simulink subsystem "Baseline"  (R2024b)
settings: Solver=VariableStepAuto  StartTime=0.0  StopTime=10.0  RelTol=1e-3
undefined symbols (not defined in the file or in its folder): SimIn, SimPar
libraries: simulink_extras x23, ComponentsLib x8, libAxisTransformations x3, AdaptiveLib x1
settings Model: Creator=tbritton  LastModifiedBy=mjki1
settings SolverCC: AlgebraicLoopSolver=TrustRegion
settings OptimizationCC: ReuseModelBlockBuffer=off
settings DebuggingCC: UnconnectedInputMsg=warning  UnconnectedOutputMsg=warning  UnconnectedLineMsg=warning
settings ModelReferenceCC: EnableRefExpFcnMdlSchedulingChecks=on
settings RTWCC: GPUComputeCapability=3.5  DLArmComputeVersion=19.05

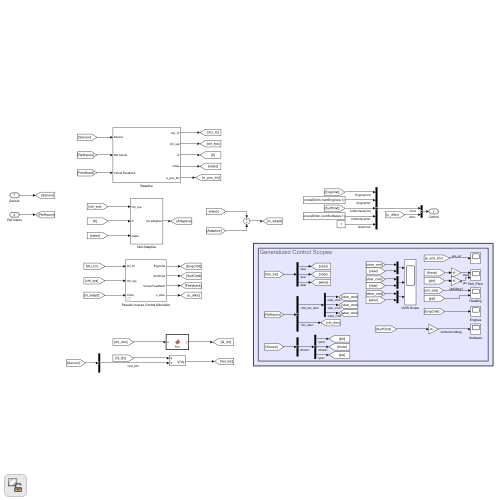
[thumbnail: Simulink's stored preview of the top-level diagram]
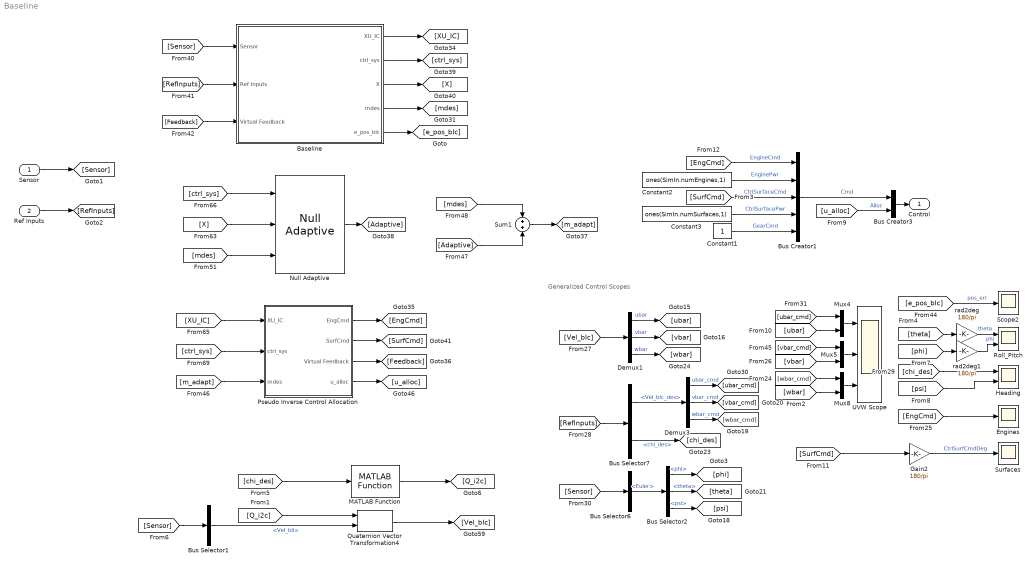
== system Baseline ==
  note: Generalized Control Scopes
  Sensor : Inport  OutDataTypeStr=Bus: SensorBus
  Ref Inputs : Inport  Port=2  OutDataTypeStr=Bus: BUS_REF_INPUT
  Baseline : Subsystem
      settings: LibrarySourceBlock=ControllersLib/Baseline
  Bus Creator1 : BusCreator  Inputs=5  OutDataTypeStr=Bus: BUS_CMD
  Bus Creator3 : BusCreator  Inputs=2
  Bus Selector1 : BusSelector  OutputSignals=Vel_bIi
  Bus Selector2 : BusSelector  OutputSignals=phi,theta,psi
  Bus Selector6 : BusSelector  OutputSignals=Euler
  Bus Selector7 : BusSelector  OutputSignals=Vel_bIc_des,chi_des
  Constant1 : Constant
  Constant2 : Constant  Value=ones(SimIn.numEngines,1)
  Constant3 : Constant  Value=ones(SimIn.numSurfaces,1)
  Demux1 : Demux  Outputs=3
  Demux3 : Demux  Outputs=3
  Engines : Scope
  Gain2 : Gain  Gain=180/pi
  Heading : Scope  NumInputPorts=2
  MATLAB Function : ComponentsLib/ConvertToControlFrame/MATLAB Function  SystemSampleTime=-1  VariantActivationTime=update diagram  AllowFlexibleInterface=on  Latency=0  AutoFrameSizeCalculation=off
      settings: SourceProductName=Components
  Mux4 : Mux  Inputs=2
  Mux5 : Mux  Inputs=2
  Mux8 : Mux  Inputs=2
  Null Adaptive : AdaptiveLib/Null Adaptive  SystemSampleTime=-1  VariantActivationTime=update diagram  AllowFlexibleInterface=on  Latency=0  AutoFrameSizeCalculation=off
      settings: SourceProductName=Adaptive Augmentation
  Pseudo Inverse Control Allocation : Subsystem  AncestorBlock=AllocatorsLib/Pseudo Inverse Control Allocation
      settings: LibrarySourceBlock=AllocatorsLib/Pseudo Inverse Control Allocation
  Quaternion Vector Transformation4 : libAxisTransformations/Quaternion Vector Transformation  n=0
  Roll_Pitch : Scope  NumInputPorts=2
  Scope2 : Scope
  Sum1 : Sum
  Surfaces : Scope
  UVW Scope : Scope  NumInputPorts=3
  rad2deg : Gain  Gain=180/pi
  rad2deg1 : Gain  Gain=180/pi
  Control : Outport  OutDataTypeStr=Bus: BUS_CONTROL  VectorParamsAs1DForOutWhenUnconnected=off
  wires:
  Baseline/5(e_pos_blc) -> [e_pos_bIc]
  Demux1/1 -> [ubar]  "ubar"
  Mux4/1 -> UVW Scope/1
  Demux3/3 -> [wbar_cmd]  "wbar_cmd"
  Mux5/1 -> UVW Scope/2
  [vbar_cmd] -> Mux5/1
  [ubar_cmd] -> Mux4/1
  [vbar] -> Mux5/2
  [SurfCmd] -> Gain2/1
  [chi_des] -> Heading/1
  [ubar] -> Mux4/2
  [Sensor] -> Bus Selector6/1
  [RefInputs] -> Bus Selector7/1
  [wbar] -> Mux8/2
  [phi] -> rad2deg1/1
  Demux3/2 -> [vbar_cmd]  "vbar_cmd"
  [e_pos_bIc] -> Scope2/1  "pos_err"
  Bus Selector6/1 -> Bus Selector2/1  "<Euler>"
  Bus Selector2/1 -> [phi]  "<phi>"
  Mux8/1 -> UVW Scope/3
  Bus Selector2/3 -> [psi]  "<psi>"
  Gain2/1 -> Surfaces/1  "CtrlSurfCmdDeg"
  [theta] -> rad2deg/1
  Bus Selector2/2 -> [theta]  "<theta>"
  [psi] -> Heading/2
  Demux1/2 -> [vbar]  "vbar"
  [EngCmd] -> Engines/1
  Bus Selector7/1 -> Demux3/1  "<Vel_bIc_des>"
  Demux3/1 -> [ubar_cmd]  "ubar_cmd"
  [Vel_bIc] -> Demux1/1
  Bus Selector7/2 -> [chi_des]  "<chi_des>"
  [wbar_cmd] -> Mux8/1
  Demux1/3 -> [wbar]  "wbar"
  [Sensor] -> Bus Selector1/1
  MATLAB Function/1 -> [Q_i2c]
  Quaternion Vector Transformation4/1 -> [Vel_bIc]
  [chi_des] -> MATLAB Function/1
  [Q_i2c] -> Quaternion Vector Transformation4/1
  Bus Selector1/1 -> Quaternion Vector Transformation4/2  "<Vel_bIi>"
  [ctrl_sys] -> Pseudo Inverse Control Allocation/2(ctrl_sys)
  [XU_IC] -> Pseudo Inverse Control Allocation/1(XU_IC)
  Pseudo Inverse Control Allocation/4(u_alloc) -> [u_alloc]
  Pseudo Inverse Control Allocation/2(SurfCmd) -> [SurfCmd]
  [Adaptive] -> Sum1/2
  [mdes] -> Sum1/1
  Sum1/1 -> [m_adapt]
  Baseline/3(X) -> [X]
  Baseline/2(ctrl_sys) -> [ctrl_sys]
  Null Adaptive/1 -> [Adaptive]
  [X] -> Null Adaptive/2
  [mdes] -> Null Adaptive/3
  [ctrl_sys] -> Null Adaptive/1
  Pseudo Inverse Control Allocation/1(EngCmd) -> [EngCmd]
  Baseline/1(XU_IC) -> [XU_IC]
  Pseudo Inverse Control Allocation/3(Virtual Feedback) -> [Feedback]
  [m_adapt] -> Pseudo Inverse Control Allocation/3(mdes)
  Baseline/4(mdes) -> [mdes]
  [Feedback] -> Baseline/3(Virtual Feedback)
  [RefInputs] -> Baseline/2(Ref Inputs)
  [Sensor] -> Baseline/1(Sensor)
  Constant3/1 -> Bus Creator1/4  "CtrlSurfacePwr"
  Constant2/1 -> Bus Creator1/2  "EnginePwr"
  [EngCmd] -> Bus Creator1/1  "EngineCmd"
  Sensor/1 -> [Sensor]
  Bus Creator1/1 -> Bus Creator3/1  "Cmd"
  [SurfCmd] -> Bus Creator1/3  "CtrlSurfaceCmd"
  Constant1/1 -> Bus Creator1/5  "GearCmd"
  Bus Creator3/1 -> Control/1
  [u_alloc] -> Bus Creator3/2  "Alloc"
  Ref Inputs/1 -> [RefInputs]
  rad2deg/1 -> Roll_Pitch/1  "theta"
  rad2deg1/1 -> Roll_Pitch/2  "phi"

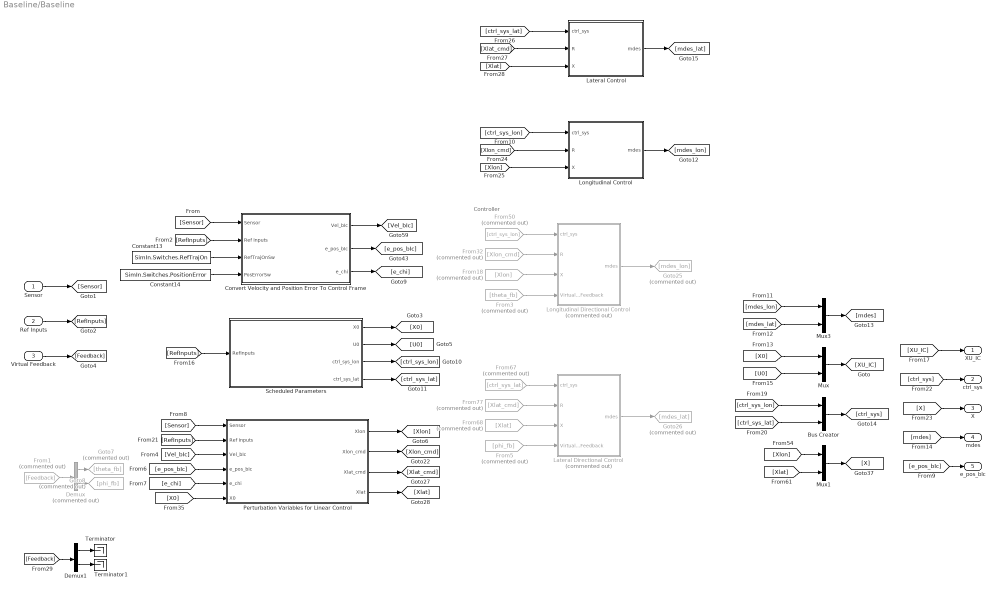
== system Baseline/Baseline ==
  note: Controller
  Sensor : Inport  OutDataTypeStr=Bus: SensorBus
  Ref Inputs : Inport  Port=2  OutDataTypeStr=Bus: BUS_REF_INPUT
  Virtual Feedback : Inport  Port=3
  Bus Creator : BusCreator  Inputs=2
  Constant13 : Constant  Value=SimIn.Switches.RefTrajOn
  Constant14 : Constant  Value=SimIn.Switches.PositionError
  Convert Velocity and Position Error To Control Frame : Subsystem  AncestorBlock=ComponentsLib/ConvertToControlFrame
  Demux : Demux  Commented=on  Outputs=2
  Demux1 : Demux  Outputs=2
  From1 : From  Commented=on  GotoTag=Feedback
  From18 : From  Commented=on  GotoTag=Xlon
  From3 : From  Commented=on  GotoTag=theta_fb
  From32 : From  Commented=on  GotoTag=Xlon_cmd
  From5 : From  Commented=on  GotoTag=phi_fb
  From50 : From  Commented=on  GotoTag=ctrl_sys_lon
  From67 : From  Commented=on  GotoTag=ctrl_sys_lat
  From68 : From  Commented=on  GotoTag=Xlat
  From77 : From  Commented=on  GotoTag=Xlat_cmd
  Goto25 : Goto  Commented=on  GotoTag=mdes_lon
  Goto26 : Goto  Commented=on  GotoTag=mdes_lat
  Goto7 : Goto  Commented=on  GotoTag=theta_fb
  Goto8 : Goto  Commented=on  GotoTag=phi_fb
  Lateral Control : Subsystem
  Lateral Directional Control : Subsystem  Commented=on  AncestorBlock=ComponentsLib/DirectionalControl
  Longitudinal Control : Subsystem
  Longitudinal Directional Control : Subsystem  Commented=on  AncestorBlock=ComponentsLib/DirectionalControl
      settings: LibrarySourceBlock=ComponentsLib/DirectionalControl
  Mux : Mux  Inputs=2
  Mux1 : Mux  Inputs=2
  Mux3 : Mux  Inputs=2
  Perturbation Variables for Linear Control : Subsystem  AncestorBlock=ComponentsLib/ComputePerturbationVariables
  Scheduled Parameters : Subsystem  AncestorBlock=ComponentsLib/FeedbackScheduling
      settings: LibrarySourceBlock=ComponentsLib/FeedbackScheduling
  Terminator : Terminator
  Terminator1 : Terminator
  XU_IC : Outport
  ctrl_sys : Outport  Port=2
  X : Outport  Port=3
  mdes : Outport  Port=4
  e_pos_blc : Outport  Port=5
  wires:
  [ctrl_sys_lat] -> Lateral Control/1(ctrl_sys)
  [Xlat] -> Lateral Control/3(X)
  [Xlat_cmd] -> Lateral Control/2(R)
  Lateral Control/1(mdes) -> [mdes_lat]
  Longitudinal Control/1(mdes) -> [mdes_lon]
  [Xlon] -> Longitudinal Control/3(X)
  [Xlon_cmd] -> Longitudinal Control/2(R)
  [ctrl_sys_lon] -> Longitudinal Control/1(ctrl_sys)
  [X] -> X/1
  [Xlat] -> Mux1/2
  [Xlon] -> Mux1/1
  Mux1/1 -> [X]
  [ctrl_sys] -> ctrl_sys/1
  Bus Creator/1 -> [ctrl_sys]
  [ctrl_sys_lat] -> Bus Creator/2
  [ctrl_sys_lon] -> Bus Creator/1
  [XU_IC] -> XU_IC/1
  Mux/1 -> [XU_IC]
  [U0] -> Mux/2
  [X0] -> Mux/1
  [mdes] -> mdes/1
  Mux3/1 -> [mdes]
  [mdes_lon] -> Mux3/1
  From5/1 -> Lateral Directional Control/4(Virtual Feedback)
  From3/1 -> Longitudinal Directional Control/4(Virtual Feedback)
  Demux/1 -> Goto7/1
  Demux/2 -> Goto8/1
  From1/1 -> Demux/1
  Virtual Feedback/1 -> [Feedback]
  From77/1 -> Lateral Directional Control/2(R)
  From18/1 -> Longitudinal Directional Control/3(X)
  From68/1 -> Lateral Directional Control/3(X)
  Longitudinal Directional Control/1(mdes) -> Goto25/1
  From50/1 -> Longitudinal Directional Control/1(ctrl_sys)
  From67/1 -> Lateral Directional Control/1(ctrl_sys)
  Lateral Directional Control/1(mdes) -> Goto26/1
  From32/1 -> Longitudinal Directional Control/2(R)
  Scheduled Parameters/4(ctrl_sys_lat) -> [ctrl_sys_lat]
  Scheduled Parameters/2(U0) -> [U0]
  [e_chi] -> Perturbation Variables for Linear Control/5(e_chi)
  Constant14/1 -> Convert Velocity and Position Error To Control Frame/4(PosErrorSw)
  [RefInputs] -> Perturbation Variables for Linear Control/2(Ref Inputs)
  Constant13/1 -> Convert Velocity and Position Error To Control Frame/3(RefTrajOnSw)
  [Vel_bIc] -> Perturbation Variables for Linear Control/3(Vel_bIc)
  [Sensor] -> Convert Velocity and Position Error To Control Frame/1(Sensor)
  Convert Velocity and Position Error To Control Frame/3(e_chi) -> [e_chi]
  Perturbation Variables for Linear Control/2(Xlon_cmd) -> [Xlon_cmd]
  [RefInputs] -> Scheduled Parameters/1(RefInputs)
  Perturbation Variables for Linear Control/4(Xlat) -> [Xlat]
  [e_pos_bIc] -> Perturbation Variables for Linear Control/4(e_pos_bIc)
  Scheduled Parameters/3(ctrl_sys_lon) -> [ctrl_sys_lon]
  Convert Velocity and Position Error To Control Frame/2(e_pos_bIc) -> [e_pos_bIc]
  Convert Velocity and Position Error To Control Frame/1(Vel_bIc) -> [Vel_bIc]
  [RefInputs] -> Convert Velocity and Position Error To Control Frame/2(Ref Inputs)
  Ref Inputs/1 -> [RefInputs]
  Scheduled Parameters/1(X0) -> [X0]
  Sensor/1 -> [Sensor]
  Perturbation Variables for Linear Control/3(Xlat_cmd) -> [Xlat_cmd]
  [Sensor] -> Perturbation Variables for Linear Control/1(Sensor)
  Perturbation Variables for Linear Control/1(Xlon) -> [Xlon]
  [X0] -> Perturbation Variables for Linear Control/6(X0)
  [e_pos_bIc] -> e_pos_blc/1
  [mdes_lat] -> Mux3/2
  Demux1/2 -> Terminator1/1
  [Feedback] -> Demux1/1
  Demux1/1 -> Terminator/1

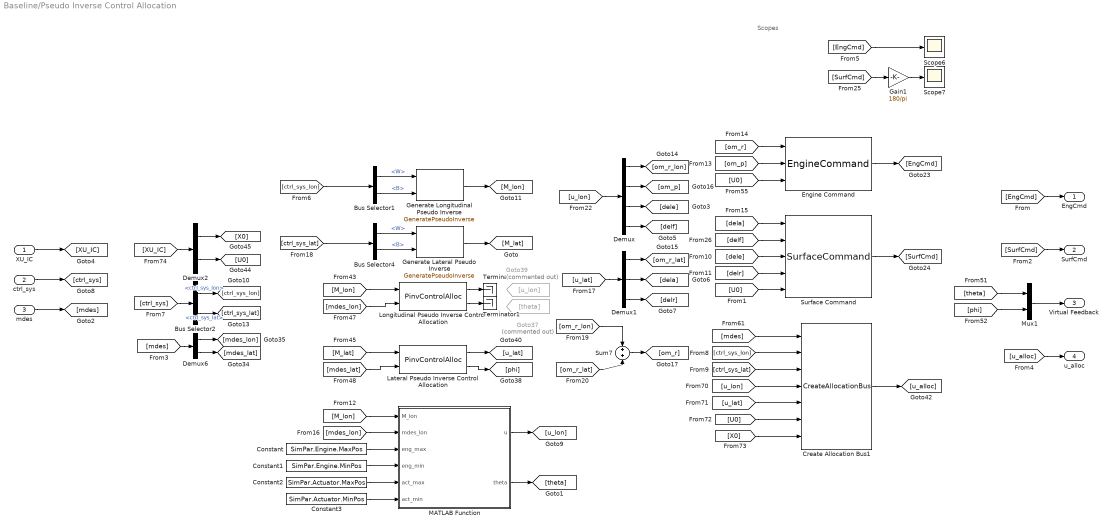
== system Baseline/Pseudo Inverse Control Allocation ==
  note: Scopes
  XU_IC : Inport
  ctrl_sys : Inport  Port=2
  mdes : Inport  Port=3
  Bus Selector1 : BusSelector  OutputSignals=W,B
  Bus Selector2 : BusSelector  OutputSignals=ctrl_sys_lon,ctrl_sys_lat
  Bus Selector4 : BusSelector  OutputSignals=W,B
  Constant : Constant  Value=SimPar.Engine.MaxPos
  Constant1 : Constant  Value=SimPar.Engine.MinPos
  Constant2 : Constant  Value=SimPar.Actuator.MaxPos
  Constant3 : Constant  Value=SimPar.Actuator.MinPos
  Create Allocation Bus1 : ComponentsLib/CreateAllocationBus  SystemSampleTime=-1  VariantActivationTime=update diagram  AllowFlexibleInterface=on  Latency=0  AutoFrameSizeCalculation=off
      settings: SourceProductName=Components
  Demux : Demux  Outputs=[8 1 1 1]
  Demux1 : Demux  Outputs=[8 1 1]
  Demux2 : Demux  Outputs=[12 13]
  Demux6 : Demux  Outputs=[3 3]
  Engine Command : ComponentsLib/EngineCommand  SystemSampleTime=-1  VariantActivationTime=update diagram  AllowFlexibleInterface=on  Latency=0  AutoFrameSizeCalculation=off
      settings: SourceProductName=Components
  Gain1 : Gain  Gain=180/pi
  Generate Lateral Pseudo Inverse : ComponentsLib/GeneratePseudoInverse  SystemSampleTime=-1  VariantActivationTime=update diagram  AllowFlexibleInterface=on  Latency=0  AutoFrameSizeCalculation=off
      settings: SourceProductName=Components
  Generate Longitudinal Pseudo Inverse : ComponentsLib/GeneratePseudoInverse  SystemSampleTime=-1  VariantActivationTime=update diagram  AllowFlexibleInterface=on  Latency=0  AutoFrameSizeCalculation=off
      settings: SourceProductName=Components
  Goto37 : Goto  Commented=on  GotoTag=theta
  Goto39 : Goto  Commented=on  GotoTag=u_lon
  Lateral Pseudo Inverse Control Allocation : ComponentsLib/PinvControlAlloc  SystemSampleTime=-1  VariantActivationTime=update diagram  AllowFlexibleInterface=on  Latency=0  AutoFrameSizeCalculation=off
      settings: SourceProductName=Components
  Longitudinal Pseudo Inverse Control Allocation : ComponentsLib/PinvControlAlloc  SystemSampleTime=-1  VariantActivationTime=update diagram  AllowFlexibleInterface=on  Latency=0  AutoFrameSizeCalculation=off
      settings: SourceProductName=Components
  MATLAB Function : MATLAB Function  TreatAsAtomicUnit=on
  Mux1 : Mux  Inputs=2
  Scope6 : Scope
  Scope7 : Scope
  Sum7 : Sum
  Surface Command : ComponentsLib/SurfaceCommand  SystemSampleTime=-1  VariantActivationTime=update diagram  AllowFlexibleInterface=on  Latency=0  AutoFrameSizeCalculation=off
      settings: SourceProductName=Components
  Terminator : Terminator
  Terminator1 : Terminator
  EngCmd : Outport
  SurfCmd : Outport  Port=2
  Virtual Feedback : Outport  Port=3
  u_alloc : Outport  Port=4
  wires:
  Constant/1 -> MATLAB Function/3(eng_max)
  Constant1/1 -> MATLAB Function/4(eng_min)
  Constant2/1 -> MATLAB Function/5(act_max)
  Constant3/1 -> MATLAB Function/6(act_min)
  MATLAB Function/2(theta) -> [theta]
  MATLAB Function/1(u) -> [u_lon]
  [mdes_lon] -> MATLAB Function/2(mdes_lon)
  [M_lon] -> MATLAB Function/1(M_lon)
  [ctrl_sys_lat] -> Create Allocation Bus1/3
  [ctrl_sys_lon] -> Create Allocation Bus1/2
  Bus Selector2/2 -> [ctrl_sys_lat]  "<ctrl_sys_lat>"
  Bus Selector2/1 -> [ctrl_sys_lon]  "<ctrl_sys_lon>"
  [ctrl_sys] -> Bus Selector2/1
  Bus Selector1/2 -> Generate Longitudinal Pseudo Inverse/2  "<B>"
  Bus Selector4/2 -> Generate Lateral Pseudo Inverse/2  "<B>"
  Generate Lateral Pseudo Inverse/1 -> [M_lat]
  Bus Selector4/1 -> Generate Lateral Pseudo Inverse/1  "<W>"
  Generate Longitudinal Pseudo Inverse/1 -> [M_lon]
  [ctrl_sys_lon] -> Bus Selector1/1
  Bus Selector1/1 -> Generate Longitudinal Pseudo Inverse/1  "<W>"
  [ctrl_sys_lat] -> Bus Selector4/1
  [EngCmd] -> Scope6/1
  [SurfCmd] -> Gain1/1
  Gain1/1 -> Scope7/1
  [u_alloc] -> u_alloc/1
  ctrl_sys/1 -> [ctrl_sys]
  XU_IC/1 -> [XU_IC]
  mdes/1 -> [mdes]
  [mdes] -> Demux6/1
  Demux6/1 -> [mdes_lon]
  Demux6/2 -> [mdes_lat]
  [mdes] -> Create Allocation Bus1/1
  Demux2/1 -> [X0]
  [X0] -> Create Allocation Bus1/7
  [XU_IC] -> Demux2/1
  [u_lat] -> Create Allocation Bus1/5
  Create Allocation Bus1/1 -> [u_alloc]
  [u_lon] -> Create Allocation Bus1/4
  [U0] -> Create Allocation Bus1/6
  Demux2/2 -> [U0]
  [SurfCmd] -> SurfCmd/1
  [EngCmd] -> EngCmd/1
  [dela] -> Surface Command/1
  [U0] -> Surface Command/5
  [om_r] -> Engine Command/1
  [om_p] -> Engine Command/2
  [delr] -> Surface Command/4
  [delf] -> Surface Command/2
  [dele] -> Surface Command/3
  [U0] -> Engine Command/3
  Surface Command/1 -> [SurfCmd]
  Engine Command/1 -> [EngCmd]
  Demux1/3 -> [delr]
  Demux/4 -> [delf]
  Demux/1 -> [om_r_lon]
  Demux1/1 -> [om_r_lat]
  Demux1/2 -> [dela]
  [u_lon] -> Demux/1
  Sum7/1 -> [om_r]
  [om_r_lon] -> Sum7/1
  [om_r_lat] -> Sum7/2
  [u_lat] -> Demux1/1
  Demux/2 -> [om_p]
  Demux/3 -> [dele]
  [M_lat] -> Lateral Pseudo Inverse Control Allocation/1
  [M_lon] -> Longitudinal Pseudo Inverse Control Allocation/1
  Mux1/1 -> Virtual Feedback/1
  Longitudinal Pseudo Inverse Control Allocation/2 -> Terminator1/1
  Lateral Pseudo Inverse Control Allocation/1 -> [u_lat]
  [mdes_lon] -> Longitudinal Pseudo Inverse Control Allocation/2
  [phi] -> Mux1/2
  [mdes_lat] -> Lateral Pseudo Inverse Control Allocation/2
  [theta] -> Mux1/1
  Longitudinal Pseudo Inverse Control Allocation/1 -> Terminator/1
  Lateral Pseudo Inverse Control Allocation/2 -> [phi]

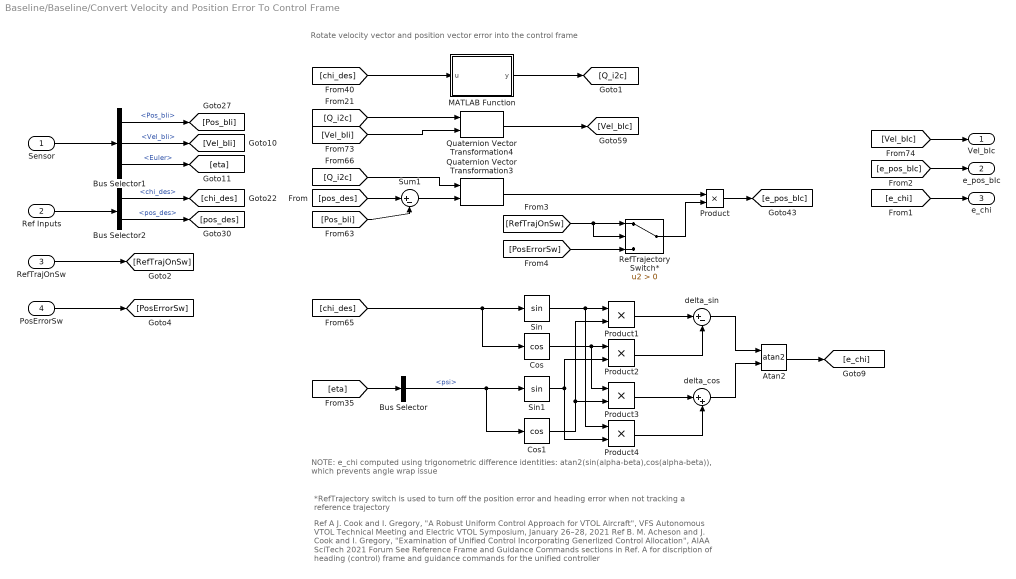
== system Baseline/Baseline/Convert Velocity and Position Error To Control Frame ==
  note: Rotate velocity vector and position vector error into the control frame
  note: Ref A
      | J. Cook and I. Gregory, "A Robust Uniform Control Approach for VTOL Aircraft", VFS Autonomous VTOL Technical Meeting and Electric VTOL Symposium, January 26–28, 2021
      |
      | Ref B.
      | M. Acheson and J. Cook and I. Gregory, "Examination of Unified Control Incorporating Generlized Control Allocation", AIAA SciTech 2021 Forum
      |
      | See Reference Frame and Guidance Commands sections in Ref. A for discription of heading (control) frame and guidance commands for the unified controller
  note: *RefTrajectory switch is used to turn off the position error and heading error when not tracking a reference trajectory
  note: NOTE: e_chi computed using trigonometric difference identities: atan2(sin(alpha-beta),cos(alpha-beta)), which prevents angle wrap issue
  Sensor : Inport  OutDataTypeStr=Bus: SensorBus
  Ref Inputs : Inport  Port=2  OutDataTypeStr=Bus: BUS_REF_INPUT
  RefTrajOnSw : Inport  Port=3
  PosErrorSw : Inport  Port=4
  Atan2 : Trigonometry  Operator=atan2
  Bus Selector : BusSelector  OutputSignals=psi
  Bus Selector1 : BusSelector  OutputSignals=Pos_bIi,Vel_bIi,Euler
  Bus Selector2 : BusSelector  OutputSignals=chi_des,pos_des
  Cos : Trigonometry  Operator=cos
  Cos1 : Trigonometry  Operator=cos
  MATLAB Function : MATLAB Function  TreatAsAtomicUnit=on
  Product{,1..4} (5 alike) : Product
  Quaternion Vector Transformation3 : libAxisTransformations/Quaternion Vector Transformation  n=0
  Quaternion Vector Transformation4 : libAxisTransformations/Quaternion Vector Transformation  n=0
  RefTrajectory Switch* : Switch  Criteria=u2 > Threshold  SaturateOnIntegerOverflow=off  InputSameDT=off
  Sin : Trigonometry
  Sin1 : Trigonometry
  Sum1 : Sum  Inputs=|+-
  delta_cos : Sum  Inputs=|++
  delta_sin : Sum  Inputs=|+-
  Vel_bIc : Outport
  e_pos_bIc : Outport  Port=2
  e_chi : Outport  Port=3
  wires:
  delta_cos/1 -> Atan2/2
  delta_sin/1 -> Atan2/1
  Product4/1 -> delta_cos/2
  Product3/1 -> delta_cos/1
  Product2/1 -> delta_sin/2
  Product1/1 -> delta_sin/1
  Cos1/1 -> Product1/2, Product3/2
  Sin1/1 -> Product2/2, Product4/2
  Cos/1 -> Product2/1, Product3/1
  Sin/1 -> Product4/1, Product1/1
  Bus Selector/1 -> Sin1/1, Cos1/1  "<psi>"
  [Q_i2c] -> Quaternion Vector Transformation4/1
  [eta] -> Bus Selector/1
  [PosErrorSw] -> RefTrajectory Switch*/3
  Bus Selector1/3 -> [eta]  "<Euler>"
  MATLAB Function/1(y) -> [Q_i2c]
  Ref Inputs/1 -> Bus Selector2/1
  Product/1 -> [e_pos_bIc]
  [Q_i2c] -> Quaternion Vector Transformation3/1
  Quaternion Vector Transformation3/1 -> Product/1
  [pos_des] -> Sum1/1
  [e_chi] -> e_chi/1
  [chi_des] -> MATLAB Function/1(u)
  RefTrajectory Switch*/1 -> Product/2
  [Pos_bIi] -> Sum1/2
  [Vel_bIc] -> Vel_bIc/1
  [RefTrajOnSw] -> RefTrajectory Switch*/2, RefTrajectory Switch*/1
  Bus Selector2/2 -> [pos_des]  "<pos_des>"
  Bus Selector1/1 -> [Pos_bIi]  "<Pos_bIi>"
  Atan2/1 -> [e_chi]
  [Vel_bIi] -> Quaternion Vector Transformation4/2
  PosErrorSw/1 -> [PosErrorSw]
  Bus Selector1/2 -> [Vel_bIi]  "<Vel_bIi>"
  Bus Selector2/1 -> [chi_des]  "<chi_des>"
  RefTrajOnSw/1 -> [RefTrajOnSw]
  [e_pos_bIc] -> e_pos_bIc/1
  Sum1/1 -> Quaternion Vector Transformation3/2
  [chi_des] -> Sin/1, Cos/1
  Quaternion Vector Transformation4/1 -> [Vel_bIc]
  Sensor/1 -> Bus Selector1/1

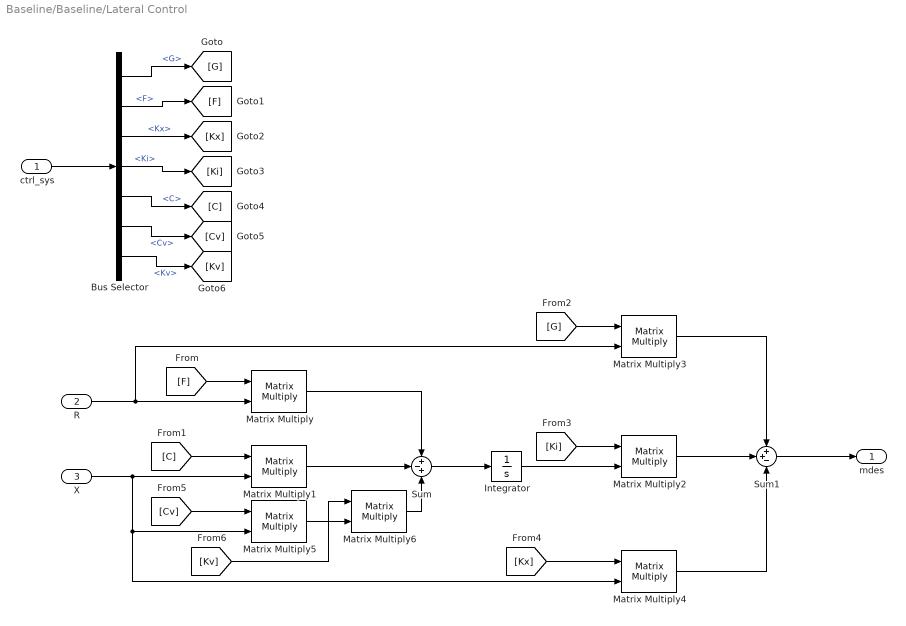
== system Baseline/Baseline/Lateral Control ==
  ctrl_sys : Inport
  R : Inport  Port=2
  X : Inport  Port=3
  Bus Selector : BusSelector  OutputSignals=G,F,Kx,Ki,C,Cv,Kv
  Integrator : Integrator
  Matrix Multiply{,1..6} (7 alike) : Product  Multiplication=Matrix(*)
  Sum : Sum  Inputs=+-+
  Sum1 : Sum  Inputs=++-
  mdes : Outport
  wires:
  Matrix Multiply6/1 -> Sum/3
  Matrix Multiply5/1 -> Matrix Multiply6/2
  [Kv] -> Matrix Multiply6/1
  [Cv] -> Matrix Multiply5/1
  Bus Selector/7 -> [Kv]  "<Kv>"
  Bus Selector/6 -> [Cv]  "<Cv>"
  Sum1/1 -> mdes/1
  Matrix Multiply4/1 -> Sum1/3
  [Kx] -> Matrix Multiply4/1
  Matrix Multiply2/1 -> Sum1/2
  Matrix Multiply3/1 -> Sum1/1
  [G] -> Matrix Multiply3/1
  Integrator/1 -> Matrix Multiply2/2
  Sum/1 -> Integrator/1
  [Ki] -> Matrix Multiply2/1
  Matrix Multiply/1 -> Sum/1
  Matrix Multiply1/1 -> Sum/2
  X/1 -> Matrix Multiply4/2, Matrix Multiply5/2, Matrix Multiply1/2
  [C] -> Matrix Multiply1/1
  [F] -> Matrix Multiply/1
  R/1 -> Matrix Multiply/2, Matrix Multiply3/2
  Bus Selector/5 -> [C]  "<C>"
  Bus Selector/4 -> [Ki]  "<Ki>"
  Bus Selector/3 -> [Kx]  "<Kx>"
  Bus Selector/2 -> [F]  "<F>"
  Bus Selector/1 -> [G]  "<G>"
  ctrl_sys/1 -> Bus Selector/1

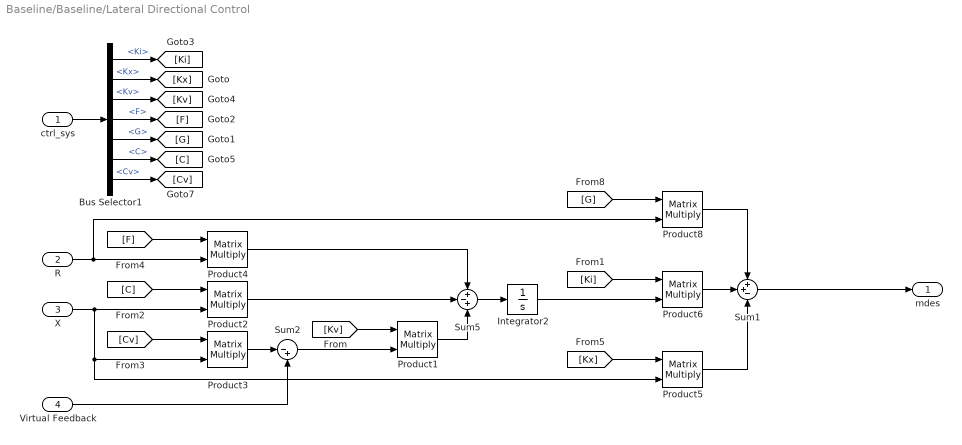
== system Baseline/Baseline/Lateral Directional Control ==
  ctrl_sys : Inport
  R : Inport  Port=2
  X : Inport  Port=3
  Virtual Feedback : Inport  Port=4
  Bus Selector1 : BusSelector  OutputSignals=Ki,Kx,Kv,F,G,C,Cv
  Integrator2 : Integrator  UpperSaturationLimit=[10 10 1]  LowerSaturationLimit=[-10 -10 -1]
  Product{1..6,8} (7 alike) : Product  Multiplication=Matrix(*)
  Sum1 : Sum  Inputs=++-
  Sum2 : Sum  Inputs=|-+
  Sum5 : Sum  Inputs=+-+
  mdes : Outport
  wires:
  Bus Selector1/1 -> [Ki]  "<Ki>"
  Bus Selector1/2 -> [Kx]  "<Kx>"
  Bus Selector1/3 -> [Kv]  "<Kv>"
  Bus Selector1/4 -> [F]  "<F>"
  Bus Selector1/5 -> [G]  "<G>"
  Bus Selector1/6 -> [C]  "<C>"
  Bus Selector1/7 -> [Cv]  "<Cv>"
  Virtual Feedback/1 -> Sum2/2
  [G] -> Product8/1
  Product8/1 -> Sum1/1
  Product4/1 -> Sum5/1
  [F] -> Product4/1
  Product5/1 -> Sum1/3
  [Kx] -> Product5/1
  Product6/1 -> Sum1/2
  [Ki] -> Product6/1
  Product1/1 -> Sum5/3
  [Kv] -> Product1/1
  Sum2/1 -> Product1/2
  Integrator2/1 -> Product6/2
  Product3/1 -> Sum2/1
  [Cv] -> Product3/1
  ctrl_sys/1 -> Bus Selector1/1
  Sum5/1 -> Integrator2/1
  R/1 -> Product4/2, Product8/2
  Product2/1 -> Sum5/2
  [C] -> Product2/1
  X/1 -> Product5/2, Product3/2, Product2/2
  Sum1/1 -> mdes/1

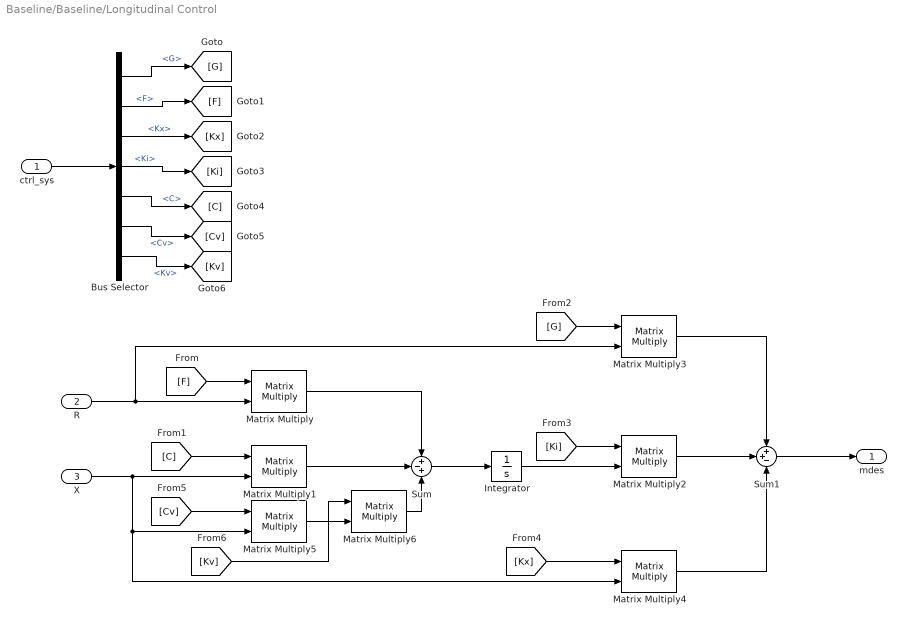
== system Baseline/Baseline/Longitudinal Control ==
  ctrl_sys : Inport
  R : Inport  Port=2
  X : Inport  Port=3
  Bus Selector : BusSelector  OutputSignals=G,F,Kx,Ki,C,Cv,Kv
  Integrator : Integrator
  Matrix Multiply{,1..6} (7 alike) : Product  Multiplication=Matrix(*)
  Sum : Sum  Inputs=+-+
  Sum1 : Sum  Inputs=++-
  mdes : Outport
  wires:
  Bus Selector/7 -> [Kv]  "<Kv>"
  Bus Selector/2 -> [F]  "<F>"
  Bus Selector/1 -> [G]  "<G>"
  [C] -> Matrix Multiply1/1
  Matrix Multiply3/1 -> Sum1/1
  Sum1/1 -> mdes/1
  [F] -> Matrix Multiply/1
  [Kv] -> Matrix Multiply6/1
  Bus Selector/5 -> [C]  "<C>"
  Sum/1 -> Integrator/1
  [G] -> Matrix Multiply3/1
  Integrator/1 -> Matrix Multiply2/2
  Matrix Multiply2/1 -> Sum1/2
  Matrix Multiply1/1 -> Sum/2
  Bus Selector/4 -> [Ki]  "<Ki>"
  Matrix Multiply6/1 -> Sum/3
  R/1 -> Matrix Multiply/2, Matrix Multiply3/2
  Matrix Multiply/1 -> Sum/1
  [Kx] -> Matrix Multiply4/1
  Matrix Multiply5/1 -> Matrix Multiply6/2
  Bus Selector/3 -> [Kx]  "<Kx>"
  X/1 -> Matrix Multiply4/2, Matrix Multiply5/2, Matrix Multiply1/2
  Matrix Multiply4/1 -> Sum1/3
  [Ki] -> Matrix Multiply2/1
  [Cv] -> Matrix Multiply5/1
  ctrl_sys/1 -> Bus Selector/1
  Bus Selector/6 -> [Cv]  "<Cv>"

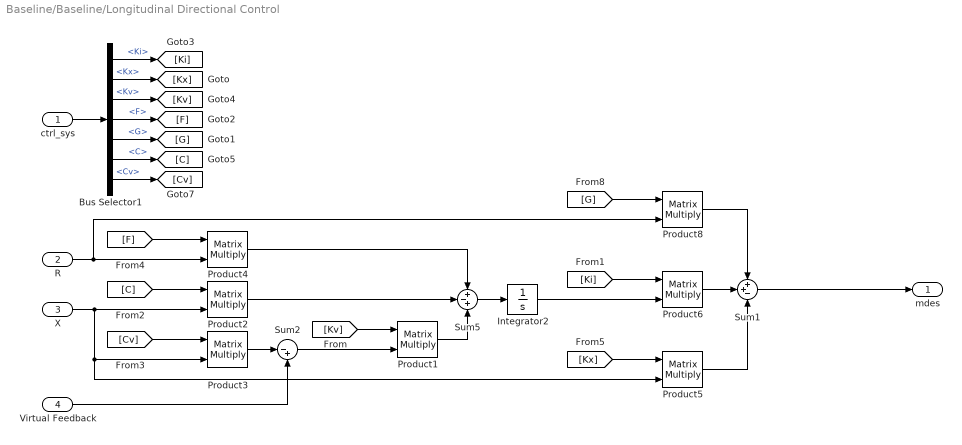
== system Baseline/Baseline/Longitudinal Directional Control ==
  ctrl_sys : Inport
  R : Inport  Port=2
  X : Inport  Port=3
  Virtual Feedback : Inport  Port=4
  Bus Selector1 : BusSelector  OutputSignals=Ki,Kx,Kv,F,G,C,Cv
  Integrator2 : Integrator  UpperSaturationLimit=[10 10 1]  LowerSaturationLimit=[-10 -10 -1]
  Product{1..6,8} (7 alike) : Product  Multiplication=Matrix(*)
  Sum1 : Sum  Inputs=++-
  Sum2 : Sum  Inputs=|-+
  Sum5 : Sum  Inputs=+-+
  mdes : Outport
  wires:
  Bus Selector1/1 -> [Ki]  "<Ki>"
  Bus Selector1/2 -> [Kx]  "<Kx>"
  Bus Selector1/3 -> [Kv]  "<Kv>"
  Bus Selector1/4 -> [F]  "<F>"
  Bus Selector1/5 -> [G]  "<G>"
  Bus Selector1/6 -> [C]  "<C>"
  Bus Selector1/7 -> [Cv]  "<Cv>"
  Virtual Feedback/1 -> Sum2/2
  [G] -> Product8/1
  Product8/1 -> Sum1/1
  Product4/1 -> Sum5/1
  [F] -> Product4/1
  Product5/1 -> Sum1/3
  [Kx] -> Product5/1
  Product6/1 -> Sum1/2
  [Ki] -> Product6/1
  Product1/1 -> Sum5/3
  [Kv] -> Product1/1
  Sum2/1 -> Product1/2
  Integrator2/1 -> Product6/2
  Product3/1 -> Sum2/1
  [Cv] -> Product3/1
  ctrl_sys/1 -> Bus Selector1/1
  Sum5/1 -> Integrator2/1
  R/1 -> Product4/2, Product8/2
  Product2/1 -> Sum5/2
  [C] -> Product2/1
  X/1 -> Product5/2, Product3/2, Product2/2
  Sum1/1 -> mdes/1

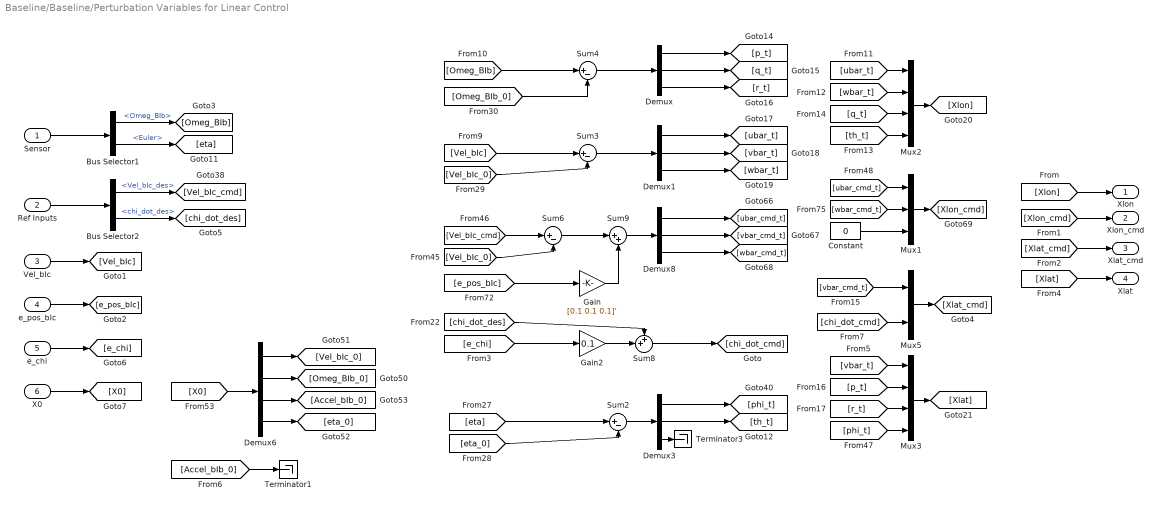
== system Baseline/Baseline/Perturbation Variables for Linear Control ==
  Sensor : Inport  OutDataTypeStr=Bus: SensorBus
  Ref Inputs : Inport  Port=2  OutDataTypeStr=Bus: BUS_REF_INPUT
  Vel_bIc : Inport  Port=3
  e_pos_bIc : Inport  Port=4
  e_chi : Inport  Port=5
  X0 : Inport  Port=6
  Bus Selector1 : BusSelector  OutputSignals=Omeg_BIb,Euler
  Bus Selector2 : BusSelector  OutputSignals=Vel_bIc_des,chi_dot_des
  Constant : Constant  Value=0
  Demux{,1,3,8} (4 alike) : Demux  Outputs=3
  Demux6 : Demux  Outputs=[3 3 3 3]
  Gain : Gain  Gain=[0.1 0.1 0.1]'
  Gain2 : Gain  Gain=0.1
  Mux1 : Mux  Inputs=3
  Mux2 : Mux
  Mux3 : Mux
  Mux5 : Mux  Inputs=2
  Sum{2..4,6} (4 alike) : Sum  Inputs=|+-
  Sum8 : Sum  Inputs=++|
  Sum9 : Sum  Inputs=|++
  Terminator1 : Terminator
  Terminator3 : Terminator
  Xlon : Outport
  Xlon_cmd : Outport  Port=2
  Xlat_cmd : Outport  Port=3
  Xlat : Outport  Port=4
  wires:
  [Accel_bIb_0] -> Terminator1/1
  X0/1 -> [X0]
  Demux6/2 -> [Omeg_BIb_0]
  Demux6/4 -> [eta_0]
  [X0] -> Demux6/1
  Demux6/3 -> [Accel_bIb_0]
  Demux6/1 -> [Vel_bIc_0]
  e_chi/1 -> [e_chi]
  e_pos_bIc/1 -> [e_pos_bIc]
  Bus Selector2/2 -> [chi_dot_des]  "<chi_dot_des>"
  Bus Selector2/1 -> [Vel_bIc_cmd]  "<Vel_bIc_des>"
  Ref Inputs/1 -> Bus Selector2/1
  Vel_bIc/1 -> [Vel_bIc]
  Bus Selector1/1 -> [Omeg_BIb]  "<Omeg_BIb>"
  Sensor/1 -> Bus Selector1/1
  Bus Selector1/2 -> [eta]  "<Euler>"
  [Xlat] -> Xlat/1
  [Xlat_cmd] -> Xlat_cmd/1
  [Xlon_cmd] -> Xlon_cmd/1
  [Xlon] -> Xlon/1
  [Omeg_BIb] -> Sum4/1
  [eta_0] -> Sum2/2
  [wbar_t] -> Mux2/2
  [ubar_cmd_t] -> Mux1/1
  Demux/2 -> [q_t]
  [th_t] -> Mux2/4
  [p_t] -> Mux3/2
  Mux3/1 -> [Xlat]
  Sum4/1 -> Demux/1
  Sum3/1 -> Demux1/1
  Demux/3 -> [r_t]
  Sum2/1 -> Demux3/1
  Demux8/2 -> [vbar_cmd_t]
  [Vel_bIc_cmd] -> Sum6/1
  Sum6/1 -> Sum9/1
  Demux8/1 -> [ubar_cmd_t]
  [phi_t] -> Mux3/4
  Constant/1 -> Mux1/3
  Demux8/3 -> [wbar_cmd_t]
  [e_pos_bIc] -> Gain/1
  [wbar_cmd_t] -> Mux1/2
  [vbar_t] -> Mux3/1
  Mux1/1 -> [Xlon_cmd]
  [chi_dot_des] -> Sum8/1
  Demux1/2 -> [vbar_t]
  [q_t] -> Mux2/3
  Mux5/1 -> [Xlat_cmd]
  [ubar_t] -> Mux2/1
  Gain/1 -> Sum9/2
  [vbar_cmd_t] -> Mux5/1
  [r_t] -> Mux3/3
  [Vel_bIc_0] -> Sum6/2
  [e_chi] -> Gain2/1
  Sum8/1 -> [chi_dot_cmd]
  Mux2/1 -> [Xlon]
  Gain2/1 -> Sum8/2
  Demux/1 -> [p_t]
  Demux1/3 -> [wbar_t]
  Demux3/1 -> [phi_t]
  Demux3/3 -> Terminator3/1
  Demux3/2 -> [th_t]
  [eta] -> Sum2/1
  Demux1/1 -> [ubar_t]
  [chi_dot_cmd] -> Mux5/2
  [Vel_bIc_0] -> Sum3/2
  [Vel_bIc] -> Sum3/1
  Sum9/1 -> Demux8/1
  [Omeg_BIb_0] -> Sum4/2

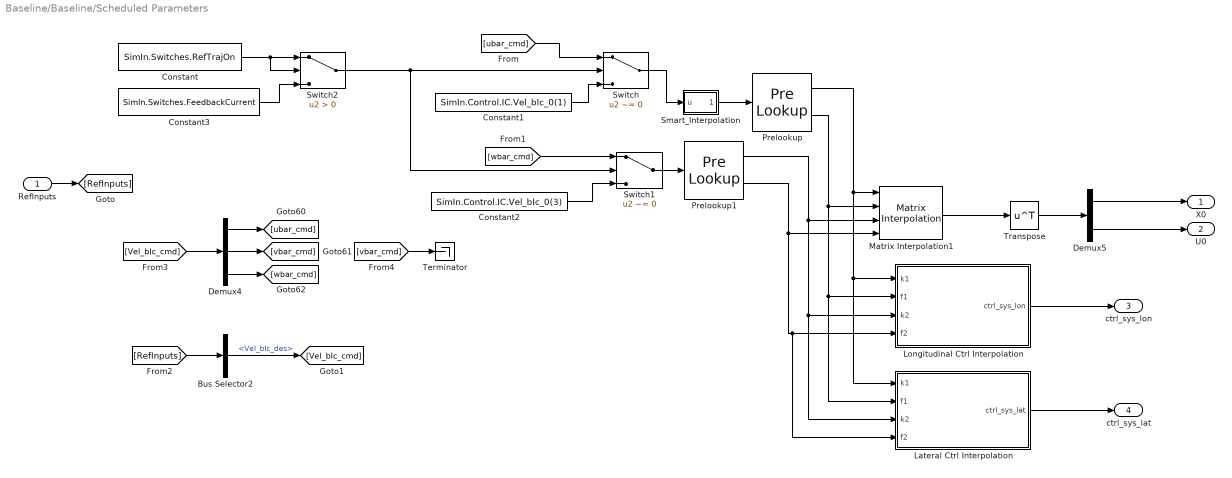
== system Baseline/Baseline/Scheduled Parameters ==
  RefInputs : Inport  OutDataTypeStr=Bus: BUS_REF_INPUT
  Bus Selector2 : BusSelector  OutputSignals=Vel_bIc_des
  Constant : Constant  Value=SimIn.Switches.RefTrajOn
  Constant1 : Constant  Value=SimIn.Control.IC.Vel_bIc_0(1)
  Constant2 : Constant  Value=SimIn.Control.IC.Vel_bIc_0(3)
  Constant3 : Constant  Value=SimIn.Switches.FeedbackCurrent
  Demux4 : Demux  Outputs=3
  Demux5 : Demux  Outputs=[12 13]
  Lateral Ctrl Interpolation : Subsystem
  Longitudinal Ctrl Interpolation : Subsystem
  Matrix Interpolation1 : simulink_extras/Additional Lookup Tables/Matrix Interpolation  InterpMethod=Linear  ExtrapMethod=Clip  InterpolateDimension=2  TableData=SimIn.Control.trim.XU0_interp  SimulateUsing=Code generation
  Prelookup : PreLookup  BreakpointsData=SimIn.Control.trim.UH
  Prelookup1 : PreLookup  BreakpointsData=SimIn.Control.trim.WH
  Smart_Interpolation : MATLAB Function  TreatAsAtomicUnit=on
  Switch : Switch  Criteria=u2 ~= 0  SaturateOnIntegerOverflow=off  InputSameDT=off
  Switch1 : Switch  Criteria=u2 ~= 0  SaturateOnIntegerOverflow=off  InputSameDT=off
  Switch2 : Switch  Criteria=u2 > Threshold  SaturateOnIntegerOverflow=off  InputSameDT=off
  Terminator : Terminator
  Transpose : Math  Operator=transpose
  X0 : Outport
  U0 : Outport  Port=2
  ctrl_sys_lon : Outport  Port=3
  ctrl_sys_lat : Outport  Port=4
  wires:
  [wbar_cmd] -> Switch1/1
  [vbar_cmd] -> Terminator/1
  Bus Selector2/1 -> [Vel_bIc_cmd]  "<Vel_bIc_des>"
  [RefInputs] -> Bus Selector2/1
  [ubar_cmd] -> Switch/1
  RefInputs/1 -> [RefInputs]
  [Vel_bIc_cmd] -> Demux4/1
  Demux4/2 -> [vbar_cmd]
  Demux4/3 -> [wbar_cmd]
  Demux4/1 -> [ubar_cmd]
  Matrix Interpolation1/1 -> Transpose/1
  Transpose/1 -> Demux5/1
  Demux5/1 -> X0/1
  Demux5/2 -> U0/1
  Prelookup1/1 -> Longitudinal Ctrl Interpolation/3(k2), Lateral Ctrl Interpolation/3(k2), Matrix Interpolation1/3
  Prelookup1/2 -> Longitudinal Ctrl Interpolation/4(f2), Lateral Ctrl Interpolation/4(f2), Matrix Interpolation1/4
  Lateral Ctrl Interpolation/1(ctrl_sys_lat) -> ctrl_sys_lat/1
  Longitudinal Ctrl Interpolation/1(ctrl_sys_lon) -> ctrl_sys_lon/1
  Constant1/1 -> Switch/3
  Switch1/1 -> Prelookup1/1
  Constant2/1 -> Switch1/3
  Switch2/1 -> Switch1/2, Switch/2
  Constant/1 -> Switch2/1, Switch2/2
  Constant3/1 -> Switch2/3
  Switch/1 -> Smart_Interpolation/1(u)
  Smart_Interpolation/1(u_out) -> Prelookup/1
  Prelookup/2 -> Longitudinal Ctrl Interpolation/2(f1), Lateral Ctrl Interpolation/2(f1), Matrix Interpolation1/2
  Prelookup/1 -> Matrix Interpolation1/1, Longitudinal Ctrl Interpolation/1(k1), Lateral Ctrl Interpolation/1(k1)

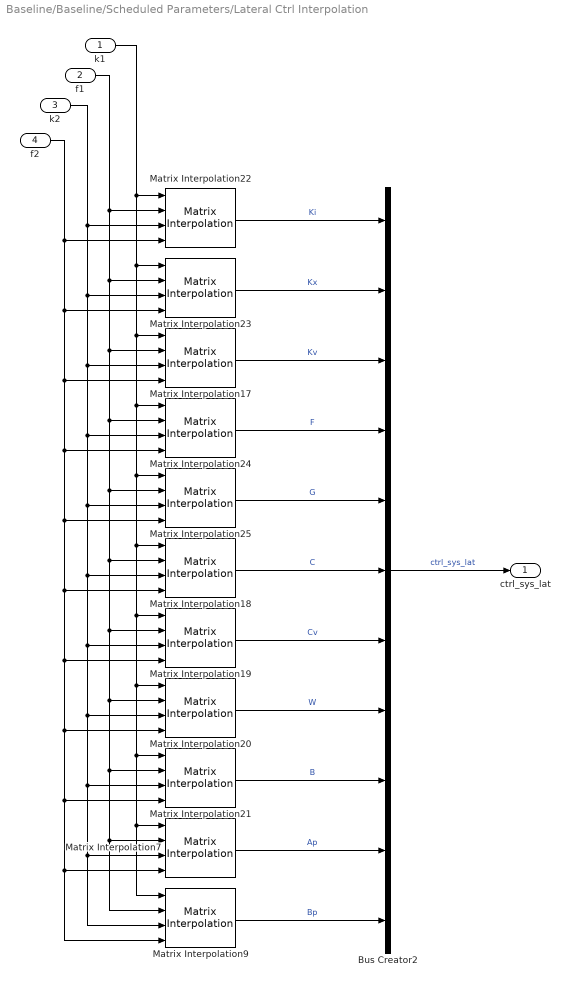
== system Baseline/Baseline/Scheduled Parameters/Lateral Ctrl Interpolation ==
  k1 : Inport
  f1 : Inport  Port=2
  k2 : Inport  Port=3
  f2 : Inport  Port=4
  Bus Creator2 : BusCreator  Inputs=11
  Matrix Interpolation17 : simulink_extras/Additional Lookup Tables/Matrix Interpolation  InterpMethod=Linear  ExtrapMethod=Clip  InterpolateDimension=2  TableData=SimIn.Control.trim.Kv_lat_interp  SimulateUsing=Code generation
  Matrix Interpolation18 : simulink_extras/Additional Lookup Tables/Matrix Interpolation  InterpMethod=Linear  ExtrapMethod=Clip  InterpolateDimension=2  TableData=SimIn.Control.trim.C_lat_interp  SimulateUsing=Code generation
  Matrix Interpolation19 : simulink_extras/Additional Lookup Tables/Matrix Interpolation  InterpMethod=Linear  ExtrapMethod=Clip  InterpolateDimension=2  TableData=SimIn.Control.trim.Cv_lat_interp  SimulateUsing=Code generation
  Matrix Interpolation20 : simulink_extras/Additional Lookup Tables/Matrix Interpolation  InterpMethod=Linear  ExtrapMethod=Clip  InterpolateDimension=2  TableData=SimIn.Control.trim.W_lat_interp  SimulateUsing=Code generation
  Matrix Interpolation21 : simulink_extras/Additional Lookup Tables/Matrix Interpolation  InterpMethod=Linear  ExtrapMethod=Clip  InterpolateDimension=2  TableData=SimIn.Control.trim.B_lat_interp  SimulateUsing=Code generation
  Matrix Interpolation22 : simulink_extras/Additional Lookup Tables/Matrix Interpolation  InterpMethod=Linear  ExtrapMethod=Clip  InterpolateDimension=2  TableData=SimIn.Control.trim.Ki_lat_interp  SimulateUsing=Code generation
  Matrix Interpolation23 : simulink_extras/Additional Lookup Tables/Matrix Interpolation  InterpMethod=Linear  ExtrapMethod=Clip  InterpolateDimension=2  TableData=SimIn.Control.trim.Kx_lat_interp  SimulateUsing=Code generation
  Matrix Interpolation24 : simulink_extras/Additional Lookup Tables/Matrix Interpolation  InterpMethod=Linear  ExtrapMethod=Clip  InterpolateDimension=2  TableData=SimIn.Control.trim.F_lat_interp  SimulateUsing=Code generation
  Matrix Interpolation25 : simulink_extras/Additional Lookup Tables/Matrix Interpolation  InterpMethod=Linear  ExtrapMethod=Clip  InterpolateDimension=2  TableData=SimIn.Control.trim.G_lat_interp  SimulateUsing=Code generation
  Matrix Interpolation7 : simulink_extras/Additional Lookup Tables/Matrix Interpolation  InterpMethod=Linear  ExtrapMethod=Clip  InterpolateDimension=2  TableData=SimIn.Control.trim.Ap_lat_interp  SimulateUsing=Code generation
  Matrix Interpolation9 : simulink_extras/Additional Lookup Tables/Matrix Interpolation  InterpMethod=Linear  ExtrapMethod=Clip  InterpolateDimension=2  TableData=SimIn.Control.trim.Bp_lat_interp  SimulateUsing=Code generation
  ctrl_sys_lat : Outport
  wires:
  k1/1 -> Matrix Interpolation22/1, Matrix Interpolation23/1, Matrix Interpolation17/1, Matrix Interpolation25/1, Matrix Interpolation18/1, Matrix Interpolation19/1, Matrix Interpolation21/1, Matrix Interpolation9/1, Matrix Interpolation7/1, Matrix Interpolation20/1, Matrix Interpolation24/1
  k2/1 -> Matrix Interpolation22/3, Matrix Interpolation23/3, Matrix Interpolation17/3, Matrix Interpolation24/3, Matrix Interpolation25/3, Matrix Interpolation18/3, Matrix Interpolation19/3, Matrix Interpolation20/3, Matrix Interpolation21/3, Matrix Interpolation7/3, Matrix Interpolation9/3
  Matrix Interpolation20/1 -> Bus Creator2/8  "W"
  f2/1 -> Matrix Interpolation22/4, Matrix Interpolation23/4, Matrix Interpolation17/4, Matrix Interpolation24/4, Matrix Interpolation25/4, Matrix Interpolation18/4, Matrix Interpolation19/4, Matrix Interpolation20/4, Matrix Interpolation21/4, Matrix Interpolation7/4, Matrix Interpolation9/4
  f1/1 -> Matrix Interpolation22/2, Matrix Interpolation23/2, Matrix Interpolation17/2, Matrix Interpolation24/2, Matrix Interpolation25/2, Matrix Interpolation18/2, Matrix Interpolation19/2, Matrix Interpolation20/2, Matrix Interpolation21/2, Matrix Interpolation7/2, Matrix Interpolation9/2
  Matrix Interpolation22/1 -> Bus Creator2/1  "Ki"
  Matrix Interpolation17/1 -> Bus Creator2/3  "Kv"
  Matrix Interpolation18/1 -> Bus Creator2/6  "C"
  Matrix Interpolation19/1 -> Bus Creator2/7  "Cv"
  Matrix Interpolation23/1 -> Bus Creator2/2  "Kx"
  Matrix Interpolation9/1 -> Bus Creator2/11  "Bp"
  Matrix Interpolation25/1 -> Bus Creator2/5  "G"
  Matrix Interpolation24/1 -> Bus Creator2/4  "F"
  Matrix Interpolation21/1 -> Bus Creator2/9  "B"
  Matrix Interpolation7/1 -> Bus Creator2/10  "Ap"
  Bus Creator2/1 -> ctrl_sys_lat/1  "ctrl_sys_lat"

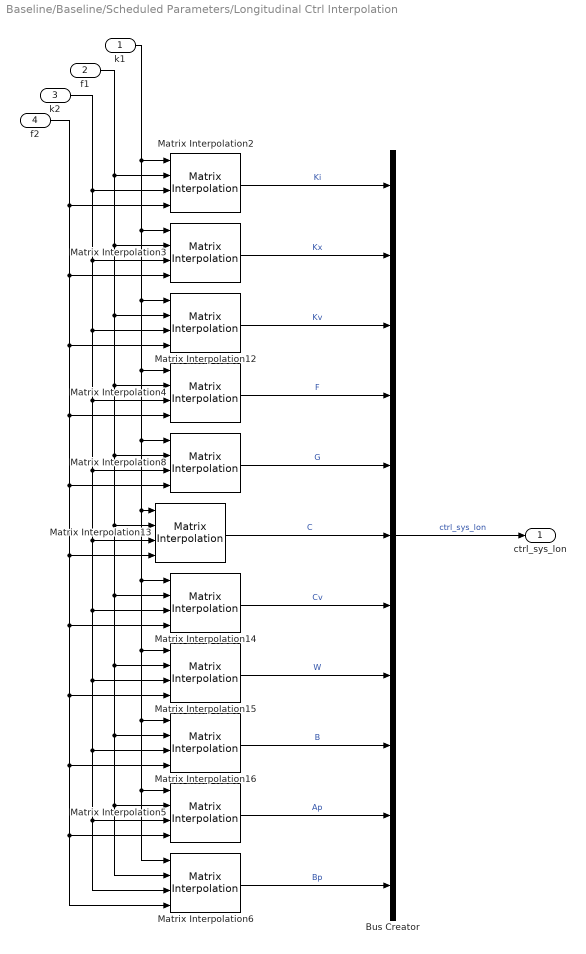
== system Baseline/Baseline/Scheduled Parameters/Longitudinal Ctrl Interpolation ==
  k1 : Inport
  f1 : Inport  Port=2
  k2 : Inport  Port=3
  f2 : Inport  Port=4
  Bus Creator : BusCreator  Inputs=11
  Matrix Interpolation12 : simulink_extras/Additional Lookup Tables/Matrix Interpolation  InterpMethod=Linear  ExtrapMethod=Clip  InterpolateDimension=2  TableData=SimIn.Control.trim.Kv_lon_interp  SimulateUsing=Code generation
  Matrix Interpolation13 : simulink_extras/Additional Lookup Tables/Matrix Interpolation  InterpMethod=Linear  ExtrapMethod=Clip  InterpolateDimension=2  TableData=SimIn.Control.trim.C_lon_interp  SimulateUsing=Code generation
  Matrix Interpolation14 : simulink_extras/Additional Lookup Tables/Matrix Interpolation  InterpMethod=Linear  ExtrapMethod=Clip  InterpolateDimension=2  TableData=SimIn.Control.trim.Cv_lon_interp  SimulateUsing=Code generation
  Matrix Interpolation15 : simulink_extras/Additional Lookup Tables/Matrix Interpolation  InterpMethod=Linear  ExtrapMethod=Clip  InterpolateDimension=2  TableData=SimIn.Control.trim.W_lon_interp  SimulateUsing=Code generation
  Matrix Interpolation16 : simulink_extras/Additional Lookup Tables/Matrix Interpolation  InterpMethod=Linear  ExtrapMethod=Clip  InterpolateDimension=2  TableData=SimIn.Control.trim.B_lon_interp  SimulateUsing=Code generation
  Matrix Interpolation2 : simulink_extras/Additional Lookup Tables/Matrix Interpolation  InterpMethod=Linear  ExtrapMethod=Clip  InterpolateDimension=2  TableData=SimIn.Control.trim.Ki_lon_interp  SimulateUsing=Code generation
  Matrix Interpolation3 : simulink_extras/Additional Lookup Tables/Matrix Interpolation  InterpMethod=Linear  ExtrapMethod=Clip  InterpolateDimension=2  TableData=SimIn.Control.trim.Kx_lon_interp  SimulateUsing=Code generation
  Matrix Interpolation4 : simulink_extras/Additional Lookup Tables/Matrix Interpolation  InterpMethod=Linear  ExtrapMethod=Clip  InterpolateDimension=2  TableData=SimIn.Control.trim.F_lon_interp  SimulateUsing=Code generation
  Matrix Interpolation5 : simulink_extras/Additional Lookup Tables/Matrix Interpolation  InterpMethod=Linear  ExtrapMethod=Clip  InterpolateDimension=2  TableData=SimIn.Control.trim.Ap_lon_interp  SimulateUsing=Code generation
  Matrix Interpolation6 : simulink_extras/Additional Lookup Tables/Matrix Interpolation  InterpMethod=Linear  ExtrapMethod=Clip  InterpolateDimension=2  TableData=SimIn.Control.trim.Bp_lon_interp  SimulateUsing=Code generation
  Matrix Interpolation8 : simulink_extras/Additional Lookup Tables/Matrix Interpolation  InterpMethod=Linear  ExtrapMethod=Clip  InterpolateDimension=2  TableData=SimIn.Control.trim.G_lon_interp  SimulateUsing=Code generation
  ctrl_sys_lon : Outport
  wires:
  f1/1 -> Matrix Interpolation2/2, Matrix Interpolation3/2, Matrix Interpolation12/2, Matrix Interpolation4/2, Matrix Interpolation8/2, Matrix Interpolation13/2, Matrix Interpolation14/2, Matrix Interpolation15/2, Matrix Interpolation16/2, Matrix Interpolation5/2, Matrix Interpolation6/2
  Matrix Interpolation6/1 -> Bus Creator/11  "Bp"
  k2/1 -> Matrix Interpolation2/3, Matrix Interpolation3/3, Matrix Interpolation12/3, Matrix Interpolation4/3, Matrix Interpolation8/3, Matrix Interpolation13/3, Matrix Interpolation14/3, Matrix Interpolation15/3, Matrix Interpolation16/3, Matrix Interpolation5/3, Matrix Interpolation6/3
  k1/1 -> Matrix Interpolation2/1, Matrix Interpolation3/1, Matrix Interpolation12/1, Matrix Interpolation4/1, Matrix Interpolation8/1, Matrix Interpolation13/1, Matrix Interpolation14/1, Matrix Interpolation15/1, Matrix Interpolation5/1, Matrix Interpolation6/1, Matrix Interpolation16/1
  Matrix Interpolation3/1 -> Bus Creator/2  "Kx"
  Matrix Interpolation13/1 -> Bus Creator/6  "C"
  Matrix Interpolation8/1 -> Bus Creator/5  "G"
  Matrix Interpolation16/1 -> Bus Creator/9  "B"
  Matrix Interpolation2/1 -> Bus Creator/1  "Ki"
  Matrix Interpolation14/1 -> Bus Creator/7  "Cv"
  Matrix Interpolation4/1 -> Bus Creator/4  "F"
  Matrix Interpolation5/1 -> Bus Creator/10  "Ap"
  Matrix Interpolation15/1 -> Bus Creator/8  "W"
  Matrix Interpolation12/1 -> Bus Creator/3  "Kv"
  Bus Creator/1 -> ctrl_sys_lon/1  "ctrl_sys_lon"
  f2/1 -> Matrix Interpolation2/4, Matrix Interpolation3/4, Matrix Interpolation12/4, Matrix Interpolation4/4, Matrix Interpolation8/4, Matrix Interpolation13/4, Matrix Interpolation14/4, Matrix Interpolation15/4, Matrix Interpolation16/4, Matrix Interpolation5/4, Matrix Interpolation6/4

== matlab function Baseline/Scheduled Parameters/Smart_Interpolation ==
  data: u input; u_out output
function u_out = fcn(u)

% This function is used to limit interpolation for three portions of the
% flight envelope: 1) Below zero knots, 2) After the end of transition
% (90 kts) and before cruise (100 knots) and 3) above the last trim map
% point (130 knots)

ft2kts = 0.3048/1852.0*3600; % Conversion factor of ft/sec to knots (derived from setUnits values)
kts2ft = 1/ft2kts; % Conversion factor from knots to ft/sec
if u < 0* kts2ft; % SimIn.Control.trim.UH(1)
    u_out = 0*kts2ft; % SimIn.Control.trim.UH(1);
% elseif u>90*kts2ft && u<100*kts2ft
%     u_out = 100*kts2ft;
elseif u>130*kts2ft % SimIn.Control.trim.UH(end)
    u_out = 130*kts2ft; % SimIn.Control.trim.UH(end)
else
    u_out = u;
end

== matlab function Baseline/Pseudo Inverse Control Allocation/MATLAB Function ==
  data: M_lon input; u output; mdes_lon input; theta output; eng_max input; eng_min input; act_max input; act_min input
function [u, theta] = Limited_Allocation(M_lon, mdes_lon, eng_max, eng_min, act_max, act_min)

[u, theta] = Limited_Long_Cont_Alloc(M_lon, mdes_lon, eng_max, eng_min, act_max, act_min);

== matlab function Baseline/Convert Velocity and Position Error To Control Frame/MATLAB Function ==
  data: u input; y output double size=[4,1]
function y = fcn(u)

s = cos(u/2);
v = sin(u/2);
y = [s, 0*v, 0*v, v]';
